simulink model "hw4q1d"  (Simulink 10.0)
settings: Solver=FixedStepAuto  StartTime=0.0  StopTime=20  FixedStep=0.01  RelTol=1e-3
libraries: slident x3
settings Model: Creator=axs2437  LastModifiedBy=axs2437
settings DataIOCC: SaveFormat=Dataset
settings OptimizationCC: LifeSpan=auto
settings DebuggingCC: UnderspecifiedInitializationDetection=Simplified  MergeDetectMultiDrivingBlocksExec=error  SFUnexpectedBacktrackingDiag=error  SFNoUnconditionalDefaultTransitionDiag=error  SFExecutionAtInitializationDiag=warning  ArithmeticOperatorsInVariantConditions=error
settings HardwareCC: ProdBitPerPointer=64  ProdBitPerSizeT=64  ProdBitPerPtrDiffT=64  ProdLargestAtomicFloat=Float  ProdIntDivRoundTo=Zero  ProdEndianess=LittleEndian  ProdWordSize=64  ProdHWDeviceType=Intel->x86-64 (Windows64)
settings ModelReferenceCC: PropagateSignalLabelsOutOfModel=on
settings SFSimCC: SimUseLocalCustomCode=on  CustomCodeUndefinedFunction=FilterOut
settings RTWCC: RTWUseLocalCustomCode=on
settings CodeAppCC: StateflowObjectComments=off
settings GRTTargetCC: TargetLangStandard=C99 (ISO)  CombineOutputUpdateFcns=on  GRTInterface=off
settings ConfigComp: CovMetricSettings=dwe  CovHtmlReporting=off  CovSaveCumulativeToWorkspaceVar=off  CovSaveSingleToWorkspaceVar=off

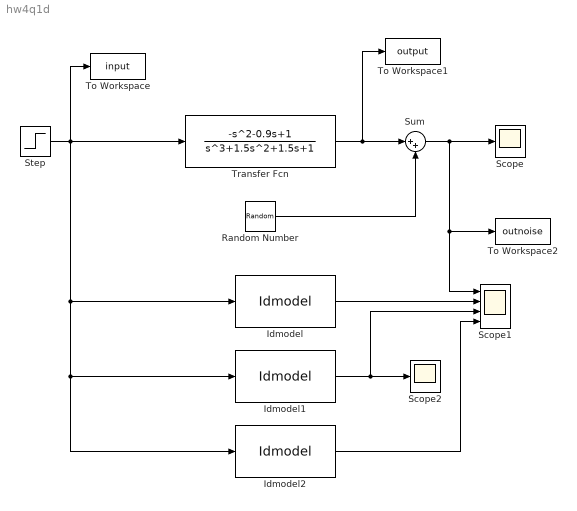
== system hw4q1d ==
  Idmodel : slident/Models/Idmodel  sys=arx_n_321  IC=0  noi=off  seed=[]
      settings: SourceProductName=System Identification Toolbox  SourceProductBaseCode=ID
  Idmodel1 : slident/Models/Idmodel  sys=arx_n_541  IC=0  noi=off  seed=[]
      settings: SourceProductName=System Identification Toolbox  SourceProductBaseCode=ID
  Idmodel2 : slident/Models/Idmodel  sys=arx_n_11101  IC=0  noi=off  seed=[]
      settings: SourceProductName=System Identification Toolbox  SourceProductBaseCode=ID
  Random Number : RandomNumber  Variance=0.001  SampleTime=0.01
  Scope : Scope
  Scope1 : Scope  NumInputPorts=4
  Scope2 : Scope
  Step : Step  SampleTime=0.01
  Sum : Sum  Inputs=|++
  To Workspace : ToWorkspace  VariableName=input  SampleTime=-1
  To Workspace1 : ToWorkspace  VariableName=output  SampleTime=-1
  To Workspace2 : ToWorkspace  VariableName=outnoise  SampleTime=-1
  Transfer Fcn : TransferFcn  Numerator=[-1 -0.9 1]  Denominator=[1 1.5 1.5 1]
  wires:
  Step/1 -> Idmodel2/1, Idmodel1/1, Idmodel/1, Transfer Fcn/1, To Workspace/1
  Transfer Fcn/1 -> Sum/1, To Workspace1/1
  Random Number/1 -> Sum/2
  Sum/1 -> Scope1/1, To Workspace2/1, Scope/1
  Idmodel/1 -> Scope1/2
  Idmodel1/1 -> Scope2/1, Scope1/3
  Idmodel2/1 -> Scope1/4
